simulink model "pointmassim"  (R2014b)
settings: Solver=ode45  StartTime=0.0  StopTime=20  RelTol=1e-3
values from neighbouring files (symbols this model uses):
  delay = del(a)    [PlantParams.m]
  h = 1/20    (= 0.05)    [PlantParams.m]
libraries: simulink x4
settings Model: Creator=mlab-retro  LastModifiedBy=mlab-retro

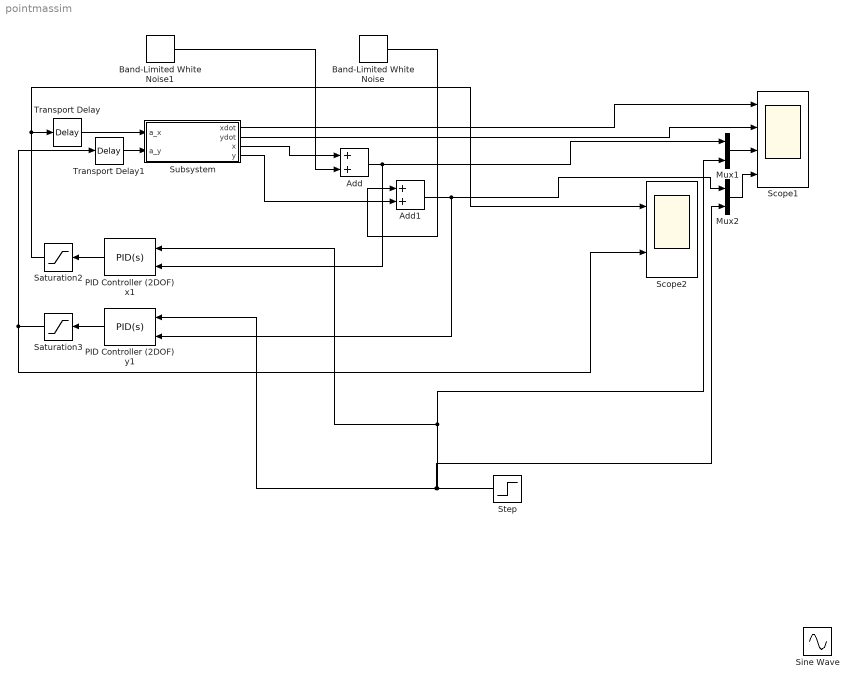
== system pointmassim ==
  Add : Sum
  Add1 : Sum
  Band-Limited White Noise : simulink/Sources/Band-Limited White Noise  Cov=est_error  Ts=h  seed=[341]
  Band-Limited White Noise1 : simulink/Sources/Band-Limited White Noise  Cov=est_error  Ts=h  seed=[23341]
  Mux1 : Mux  Inputs=2
  Mux2 : Mux  Inputs=2
  PID Controller (2DOF) x1 : simulink/Continuous/PID Controller (2DOF)  Controller=PID  TimeDomain=Continuous-time  SampleTime=-1  IntegratorMethod=Forward Euler  FilterMethod=Forward Euler  Form=Parallel  P=2  I=1  D=1  N=100  b=1  c=1  InitialConditionSource=internal  InitialConditionForIntegrator=0  InitialConditionForFilter=0  ExternalReset=none  LimitOutput=off  UpperSaturationLimit=inf  LowerSaturationLimit=-inf  LinearizeAsGain=on  AntiWindupMode=none  Kb=1  TrackingMode=off  Kt=1  PParamMin=[]  PParamMax=[]  IParamMin=[]  IParamMax=[]  DParamMin=[]  DParamMax=[]  NParamMin=[]  NParamMax=[]  bParamMin=[]  bParamMax=[]  cParamMin=[]  cParamMax=[]  KbParamMin=[]  KbParamMax=[]  KtParamMin=[]  KtParamMax=[]  POutMin=[]  POutMax=[]  IOutMin=[]  IOutMax=[]  DOutMin=[]  DOutMax=[]  NOutMin=[]  NOutMax=[]  bOutMin=[]  bOutMax=[]  cOutMin=[]  cOutMax=[]  KbOutMin=[]  KbOutMax=[]  KtOutMin=[]  KtOutMax=[]  IntegratorOutMin=[]  IntegratorOutMax=[]  FilterOutMin=[]  FilterOutMax=[]  SumOutMin=[]  SumOutMax=[]  Sum1OutMin=[]  Sum1OutMax=[]  Sum2OutMin=[]  Sum2OutMax=[]  Sum3OutMin=[]  Sum3OutMax=[]  SumI1OutMin=[]  SumI1OutMax=[]  SumI2OutMin=[]  SumI2OutMax=[]  SumI3OutMin=[]  SumI3OutMax=[]  SumDOutMin=[]  SumDOutMax=[]  SaturationOutMin=[]  SaturationOutMax=[]  IntegratorContinuousStateAttributes=''  IntegratorStateMustResolveToSignalObject=off  IntegratorRTWStateStorageClass=Auto  FilterContinuousStateAttributes=''  FilterStateMustResolveToSignalObject=off  FilterRTWStateStorageClass=Auto  DifferentiatorICPrevScaledInput=0  DifferentiatorOutMin=[]  DifferentiatorOutMax=[]  UseFilter=on
  PID Controller (2DOF) y1 : simulink/Continuous/PID Controller (2DOF)  Controller=PID  TimeDomain=Continuous-time  SampleTime=-1  IntegratorMethod=Forward Euler  FilterMethod=Forward Euler  Form=Parallel  P=2  I=1  D=1  N=100  b=1  c=1  InitialConditionSource=internal  InitialConditionForIntegrator=0  InitialConditionForFilter=0  ExternalReset=none  LimitOutput=off  UpperSaturationLimit=inf  LowerSaturationLimit=-inf  LinearizeAsGain=on  AntiWindupMode=none  Kb=1  TrackingMode=off  Kt=1  PParamMin=[]  PParamMax=[]  IParamMin=[]  IParamMax=[]  DParamMin=[]  DParamMax=[]  NParamMin=[]  NParamMax=[]  bParamMin=[]  bParamMax=[]  cParamMin=[]  cParamMax=[]  KbParamMin=[]  KbParamMax=[]  KtParamMin=[]  KtParamMax=[]  POutMin=[]  POutMax=[]  IOutMin=[]  IOutMax=[]  DOutMin=[]  DOutMax=[]  NOutMin=[]  NOutMax=[]  bOutMin=[]  bOutMax=[]  cOutMin=[]  cOutMax=[]  KbOutMin=[]  KbOutMax=[]  KtOutMin=[]  KtOutMax=[]  IntegratorOutMin=[]  IntegratorOutMax=[]  FilterOutMin=[]  FilterOutMax=[]  SumOutMin=[]  SumOutMax=[]  Sum1OutMin=[]  Sum1OutMax=[]  Sum2OutMin=[]  Sum2OutMax=[]  Sum3OutMin=[]  Sum3OutMax=[]  SumI1OutMin=[]  SumI1OutMax=[]  SumI2OutMin=[]  SumI2OutMax=[]  SumI3OutMin=[]  SumI3OutMax=[]  SumDOutMin=[]  SumDOutMax=[]  SaturationOutMin=[]  SaturationOutMax=[]  IntegratorContinuousStateAttributes=''  IntegratorStateMustResolveToSignalObject=off  IntegratorRTWStateStorageClass=Auto  FilterContinuousStateAttributes=''  FilterStateMustResolveToSignalObject=off  FilterRTWStateStorageClass=Auto  DifferentiatorICPrevScaledInput=0  DifferentiatorOutMin=[]  DifferentiatorOutMax=[]  UseFilter=on
  Saturation2 : Saturate  UpperLimit=10  LowerLimit=-10
  Saturation3 : Saturate  UpperLimit=10  LowerLimit=-10
  Scope1 : Scope  NumInputPorts=4
      settings: TimeRange=500  YMin=-5~-5~0~0  YMax=5~5~10~10  SaveName=plant
  Scope2 : Scope  NumInputPorts=2
      settings: TimeRange=10  YMin=-1~-1  YMax=1~1  SaveName=ScopeData2
  Sine Wave : Sin  Amplitude=3  SampleTime=0
  Step : Step  After=3  SampleTime=0
  Subsystem : Subsystem
  Transport Delay : TransportDelay  DelayTime=delay
  Transport Delay1 : TransportDelay  DelayTime=delay
  wires:
  PID Controller (2DOF) x1/1 -> Saturation2/1
  PID Controller (2DOF) y1/1 -> Saturation3/1
  Saturation2/1 -> Scope2/1, Transport Delay/1
  Saturation3/1 -> Transport Delay1/1, Scope2/2
  Transport Delay/1 -> Subsystem/1(a_x)
  Transport Delay1/1 -> Subsystem/2(a_y)
  Mux1/1 -> Scope1/3
  Subsystem/1(xdot) -> Scope1/1
  Subsystem/2(ydot) -> Scope1/2
  Mux2/1 -> Scope1/4
  Step/1 -> PID Controller (2DOF) y1/1, Mux2/2, Mux1/2, PID Controller (2DOF) x1/1
  Subsystem/3(x) -> Add/1
  Band-Limited White Noise1/1 -> Add/2
  Band-Limited White Noise/1 -> Add1/1
  Subsystem/4(y) -> Add1/2
  Add/1 -> PID Controller (2DOF) x1/2, Mux1/1
  Add1/1 -> PID Controller (2DOF) y1/2, Mux2/1

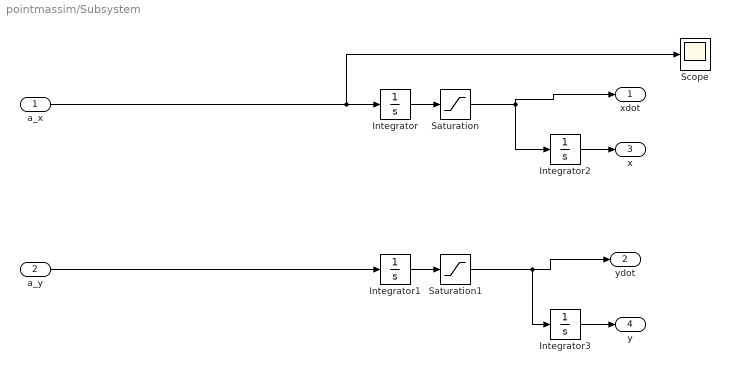
== system pointmassim/Subsystem ==
  a_x : Inport
  a_y : Inport  Port=2
  Integrator{,1..3} (4 alike) : Integrator
  Saturation : Saturate  UpperLimit=10  LowerLimit=-10
  Saturation1 : Saturate  UpperLimit=10  LowerLimit=-10
  Scope : Scope
      settings: SaveName=ScopeData3
  xdot : Outport
  ydot : Outport  Port=2
  x : Outport  Port=3
  y : Outport  Port=4
  wires:
  a_x/1 -> Scope/1, Integrator/1
  Integrator/1 -> Saturation/1
  a_y/1 -> Integrator1/1
  Integrator1/1 -> Saturation1/1
  Integrator3/1 -> y/1
  Integrator2/1 -> x/1
  Saturation/1 -> Integrator2/1, xdot/1
  Saturation1/1 -> Integrator3/1, ydot/1
